simulink model "open_phase_model"  (R2024b)
settings: Solver=ode45  StartTime=0.0  StopTime=0.1  RelTol=1e-3  EnableMultiTasking=on
values from neighbouring files (symbols this model uses):
  load_P = 40e3    (= 40000)    [main.m]
  load_P1 = load_P * 0.3    (= 12000)    [main.m]
  load_P2 = load_P * 0.3    (= 12000)    [main.m]
  load_P3 = load_P * 0.3    (= 12000)    [main.m]
undefined symbols (not defined in the file or in its folder): D1, Delta
libraries: spsFourierLib x6, spsThreePhaseVIMeasurementLib x4, spsRMSLib x4, spsParallelRLCLoadLib x3, spsSequenceAnalyzerLib x2, spsThreePhaseTransformerTwoWindingsLib x2, spsBreakerLib x1, spsThreePhaseSourceLib x1, spsGroundLib x1, spsThreePhasePISectionLineLib x1, spsThreePhaseParallelRLCLoadLib x1, spspowerguiLib x1
settings Model: Creator=jp536285  LastModifiedBy=ahmed
settings SolverCC: AlgebraicLoopSolver=TrustRegion
settings DataIOCC: LimitDataPoints=on  SaveFormat=Array  ReturnWorkspaceOutputs=off
settings OptimizationCC: LifeSpan=inf
settings DebuggingCC: UnderspecifiedInitializationDetection=Classic  MergeDetectMultiDrivingBlocksExec=none  SolverPrmCheckMsg=warning  StateNameClashWarn=warning  SFUnexpectedBacktrackingDiag=warning  SFNoUnconditionalDefaultTransitionDiag=warning  SFExecutionAtInitializationDiag=none  ArithmeticOperatorsInVariantConditions=warning
settings HardwareCC: ProdBitPerPointer=32  ProdBitPerSizeT=32  ProdBitPerPtrDiffT=32  ProdLargestAtomicFloat=None  ProdIntDivRoundTo=Undefined  ProdEndianess=Unspecified  ProdWordSize=32  ProdHWDeviceType=32-bit Generic
settings ModelReferenceCC: PropagateSignalLabelsOutOfModel=off
settings SFSimCC: SimUseLocalCustomCode=off  CustomCodeUndefinedFunction=UseInterfaceOnly
settings RTWCC: RTWUseLocalCustomCode=off  GPUComputeCapability=3.5
settings CodeAppCC: StateflowObjectComments=on
settings GRTTargetCC: TargetLangStandard=C89/C90 (ANSI)
settings ConfigComp: CovMetricSettings=dw  CovSaveCumulativeToWorkspaceVar=on  CovSaveSingleToWorkspaceVar=on  CovExternalEMLEnable=off
settings SimscapeCC: SimscapeNormalizeSystem=off  SimscapeLogOpenViewer=on

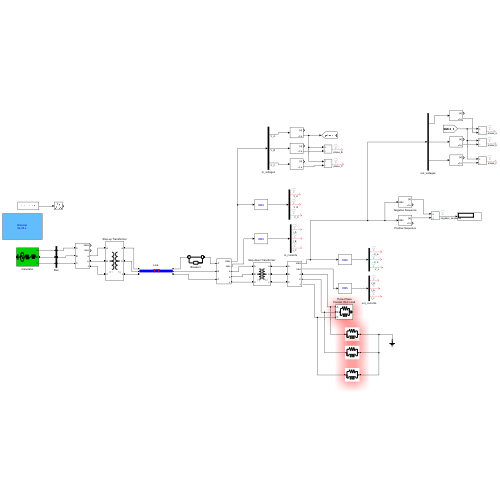
[thumbnail: Simulink's stored preview of the top-level diagram]
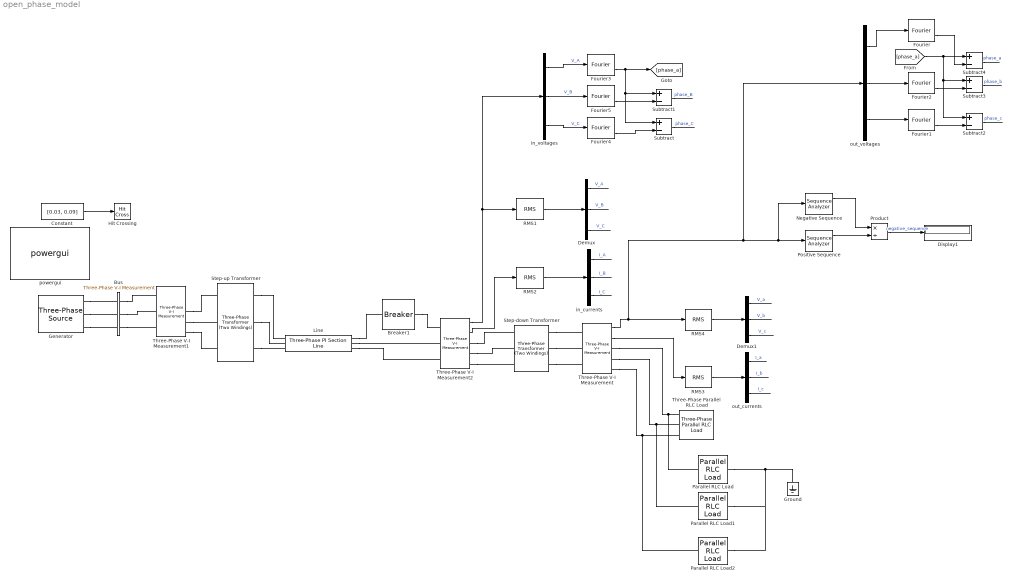
== system open_phase_model ==
  Breaker1 : spsBreakerLib/Breaker  InitialState=1  SwitchingTimes=[3/60]  External=off  BreakerResistance=0.01  SnubberResistance=1e6  SnubberCapacitance=inf  Measurements=None  MoreParameters=on  NoBreakLoop=off
  Bus : spsThreePhaseVIMeasurementLib/Three-Phase V-I Measurement  VoltageMeasurement=phase-to-ground  SetLabelV=on  LabelV=Vabc_3  Vpu=on  VpuLL=off  CurrentMeasurement=yes  SetLabelI=on  LabelI=Iabc_3  Ipu=on  Pbase=100e6  Vbase=13.8e3  OutputType=Complex  PhasorSimulation=off  PSBequivalent=0
  Constant : Constant  Value=[0.03, 0.09]
  Demux : Demux  Outputs=3
  Demux1 : Demux  Outputs=3
  Display1 : Display
  Fourier{,1..5} (6 alike) : spsFourierLib/Fourier  Freq=60  n=1  InInit=[0, 0]  Ts=0
  Generator : spsThreePhaseSourceLib/Three-Phase Source  InternalConnection=Yg  VoltagePhases=off  Voltage=13.8e3  PhaseAngle=0  Voltage_phases=[25e3 25e3 25e3]/sqrt(3)  PhaseAngles_phases=[0 -120 +120]  Frequency=60  NonIdealSource=on  SpecifyImpedance=on  Resistance=0.529  Inductance=0.0140  ShortCircuitLevel=1280e6  BaseVoltage=13.8e3  XRratio=100000  BusType=PV  Pref=85000000  Qref=0  Prefabc=[10e3, 10e3, 10e3]  Qrefabc=[0, 0, 0]  Qmin=-inf  Qmax=inf
  Ground : spsGroundLib/Ground  LConnTagsString=a
  Hit Crossing : HitCross
  Line : spsThreePhasePISectionLineLib/Three-Phase PI Section Line  LConnTagsString=a|b|c  RConnTagsString=A|B|C  Length=10  Frequency=60  Resistances=[ 0.062951 0.15737]  Inductances="[ 1.414e-3  3.53e-3]"  Capacitances=[10.47e-9 6.15e-9]  mask(Three-Phase PI Section Line){}
      mask Display:
      | % This is a new mask on top of the base mask.
      | % Use "View base mask" link below to see the base mask.
      | patch([0.0 0.0 1 1 0.0 0.0 ],[0.4 0.7 0.7 0.4 0.4 0.7],[0 0 1]);
      | patch([0.4 0.4 0.42 0.42],[0.4 0.75 0.75 0.4],[1 0 0]);
      | patch([0.38 0.38 0.57 0.57],[0.7 0.75 0.75 0.7],[1 0 0]);
      | patch([0.53 0.53 0.55 0.55],[0.4 0.75 0.75 0.4],[1 0 0]);
  Negative Sequence : spsSequenceAnalyzerLib/Sequence Analyzer  Freq=60  n=1  seq=Negative  InInit=[1, 0]  Ts=0
      settings: LibrarySourceBlock=sps_lib/Sensors and Measurements/Sequence Analyzer
  Parallel RLC Load : spsParallelRLCLoadLib/Parallel RLC Load  LConnTagsString=a  RConnTagsString=__new0  NominalVoltage=13.8e3/sqrt(3)  NominalFrequency=60  ActivePower=load_P1  InductivePower=load_P1 * 0.75  CapacitivePower=0  Setx0=off  InitialVoltage=0  SetiL0=off  InitialCurrent=0  Measurements=None  LoadType=constant Z
      settings: AttributesFormatString=\n  LibrarySourceBlock=sps_lib/Passives/Parallel RLC Load
  Parallel RLC Load1 : spsParallelRLCLoadLib/Parallel RLC Load  LConnTagsString=a  RConnTagsString=__new0  NominalVoltage=13.8e3/sqrt(3)  NominalFrequency=60  ActivePower=load_P2  InductivePower=load_P2 * 0.75  CapacitivePower=0  Setx0=off  InitialVoltage=0  SetiL0=off  InitialCurrent=0  Measurements=None  LoadType=constant Z
      settings: AttributesFormatString=\n  LibrarySourceBlock=sps_lib/Passives/Parallel RLC Load
  Parallel RLC Load2 : spsParallelRLCLoadLib/Parallel RLC Load  LConnTagsString=a  RConnTagsString=__new0  NominalVoltage=13.8e3/sqrt(3)  NominalFrequency=60  ActivePower=load_P3  InductivePower=load_P3 * 0.75  CapacitivePower=0  Setx0=off  InitialVoltage=0  SetiL0=off  InitialCurrent=0  Measurements=None  LoadType=constant Z
      settings: AttributesFormatString=\n  LibrarySourceBlock=sps_lib/Passives/Parallel RLC Load
  Positive Sequence : spsSequenceAnalyzerLib/Sequence Analyzer  Freq=60  n=1  seq=Positive  InInit=[1, 0]  Ts=0
      settings: LibrarySourceBlock=sps_lib/Sensors and Measurements/Sequence Analyzer
  Product : Product  Inputs=*/
  RMS{1..4} (4 alike) : spsRMSLib/RMS  TrueRMS=on  Freq=60  RMSInit=120  Ts=0
  Step-down Transformer : spsThreePhaseTransformerTwoWindingsLib/Three-Phase Transformer (Two Windings)  Winding1Connection=Yg  Winding2Connection=Delta (D1)  CoreType=Three-limb core (core-type)  SetSaturation=off  Hysteresis=off  DataFile='hysteresis'  SetInitialFlux=off  Measurements=None  UNITS=pu  NominalPower=[ 100e6 , 60 ]  Winding1=[ 230e3 , 1e-6 , 0 ]  Winding2=[ 13.8e3 , 1e-6, 0.0586 ]  Rm=500  Lm=500  L0=0.5  Saturation=[ 0,0 ; 0.0024,1.2 ; 1.0,1.52 ]  InitialFluxes=[ 0.8 , -0.8 , 0.7 ]  BreakLoop=off  DiscreteSolver=Trapezoidal iterative  DataType=off  TransfoNumber=1
  Step-up Transformer : spsThreePhaseTransformerTwoWindingsLib/Three-Phase Transformer (Two Windings)  Winding1Connection=Delta (D1)  Winding2Connection=Yg  CoreType=Three single-phase transformers  SetSaturation=off  Hysteresis=off  DataFile='hysteresis'  SetInitialFlux=off  Measurements=None  UNITS=pu  NominalPower=[ 100e6 , 60 ]  Winding1=[ 13.8e3 , 1e-6 , 0 ]  Winding2=[ 230e3 , 1e-6, 0.0586 ]  Rm=500  Lm=500  L0=0.5  Saturation=[ 0,0 ; 0.0024,1.2 ; 1.0,1.52 ]  InitialFluxes=[ 0.8 , -0.8 , 0.7 ]  BreakLoop=off  DiscreteSolver=Trapezoidal iterative  DataType=off  TransfoNumber=1
  Subtract{,1..4} (5 alike) : Sum  Inputs=+-
  Three-Phase Parallel  RLC Load : spsThreePhaseParallelRLCLoadLib/Three-Phase Parallel RLC Load  LConnTagsString=A|B|C  Configuration=Y (grounded)  NominalVoltage=13800  Vabc=[1e3 1e3 1e3]  Vabcp=[1e3 1e3 1e3]  NominalFrequency=60  UnbalancedPower=off  ActivePower=load_P  InductivePower=load_P * 0.75  CapacitivePower=0  Pabc=[10e3 9e3 11e3]  QLabc=[100 90 110]  QCabc=[100 90 110]  Pabcp=[10e3 9e3 11e3]  QLabcp=[100 90 110]  QCabcp=[100 90 110]  Measurements=None  LoadType=constant PQ
  Three-Phase V-I Measurement : spsThreePhaseVIMeasurementLib/Three-Phase V-I Measurement  VoltageMeasurement=phase-to-ground  SetLabelV=off  LabelV=Vabc  Vpu=off  VpuLL=off  CurrentMeasurement=yes  SetLabelI=off  LabelI=Iabc  Ipu=off  Pbase=100e6  Vbase=500e3  OutputType=Complex  PhasorSimulation=off  PSBequivalent=0
  Three-Phase V-I Measurement1 : spsThreePhaseVIMeasurementLib/Three-Phase V-I Measurement  VoltageMeasurement=phase-to-ground  SetLabelV=off  LabelV=Vabc  Vpu=off  VpuLL=off  CurrentMeasurement=yes  SetLabelI=off  LabelI=Iabc  Ipu=off  Pbase=100e6  Vbase=500e3  OutputType=Complex  PhasorSimulation=off  PSBequivalent=0
  Three-Phase V-I Measurement2 : spsThreePhaseVIMeasurementLib/Three-Phase V-I Measurement  VoltageMeasurement=phase-to-ground  SetLabelV=off  LabelV=Vabc  Vpu=off  VpuLL=off  CurrentMeasurement=yes  SetLabelI=off  LabelI=Iabc  Ipu=off  Pbase=100e6  Vbase=500e3  OutputType=Complex  PhasorSimulation=off  PSBequivalent=0
  in_currents : Demux  Outputs=3
  in_voltages : Demux  Outputs=3
  out_currents : Demux  Outputs=3
  out_voltages : Demux  Outputs=3
  powergui : spspowerguiLib/powergui  Priority=1  SimulationMode=Discrete  SampleTime=50e-6  frequency=60  Iterations=50  frequencyindice=60  Pbase=10e7  ErrMax=1e-05  UnitsV=kV  UnitsW=MW  buscounter=0  FunctionMessages=off  echomessages=off  EnableUseOfTLC=off  CurrentSourceSwitches=on  DisableSnubberDevices=off  DisableRonSwitches=off  DisableVfSwitches=off  DisplayEquations=off  AutomaticDiscreteSolvers=off  SolverType=Tustin  Interpol=off  ExternalGateDelay=off  methode=off  Ts=0  x0status=blocks  SPID=off  SwTol=0  HookPort=off  NonlinearTolerance=1e-4  nMaxIteration=100  ContinueOnMaxIteration=off  RestoreLinks=warning  ResistiveCurrentMeasurement=off  Frange=[0:2:500]  Ylog=off  Xlog=on  ShowGrid=off  save=off  variable=ZData  structure=0  ZoomFFT=off  StartTime=0.0  cycles=1  DisplayStyle=1  fundamental=60  FreqAxis=off  MaxFrequency=1000  frequencyindicesteady=1  RmsSteady=1  display=off
  wires:
  Constant/1 -> Hit Crossing/1
  Fourier/2 -> Subtract4/2
  Three-Phase V-I Measurement/2 -> RMS3/1
  Three-Phase V-I Measurement2/1 -> in_voltages/1, RMS1/1
  Fourier3/2 -> [phase_a], Subtract/1, Subtract1/1
  Three-Phase V-I Measurement2/2 -> RMS2/1
  in_voltages/2 -> Fourier5/1  "V_B"
  out_voltages/1 -> Fourier/1
  out_voltages/2 -> Fourier2/1
  in_voltages/3 -> Fourier4/1  "V_C"
  in_voltages/1 -> Fourier3/1  "V_A"
  Positive Sequence/1 -> Product/2
  RMS2/1 -> in_currents/1
  Fourier5/2 -> Subtract1/2
  Fourier4/2 -> Subtract/2
  Three-Phase V-I Measurement/1 -> Negative Sequence/1, Positive Sequence/1, out_voltages/1, RMS4/1
  Negative Sequence/1 -> Product/1
  out_voltages/3 -> Fourier1/1
  RMS3/1 -> out_currents/1
  Product/1 -> Display1/1  "negative_sequence"
  [phase_a] -> Subtract3/1, Subtract2/1, Subtract4/1
  Fourier2/2 -> Subtract3/2
  Fourier1/2 -> Subtract2/2
  RMS1/1 -> Demux/1
  Demux/1 -> ?  "V_A"
  Demux/2 -> ?  "V_B"
  Demux/3 -> ?  "V_C"
  RMS4/1 -> Demux1/1
  Demux1/1 -> ?  "V_a"
  Demux1/2 -> ?  "V_b"
  Demux1/3 -> ?  "V_c"
  out_currents/1 -> ?  "I_a"
  out_currents/2 -> ?  "I_b"
  out_currents/3 -> ?  "I_c"
  in_currents/1 -> ?  "I_A"
  in_currents/2 -> ?  "I_B"
  in_currents/3 -> ?  "I_C"
  Subtract4/1 -> ?  "phase_a"
  Subtract3/1 -> ?  "phase_b"
  Subtract2/1 -> ?  "phase_c"
  Subtract1/1 -> ?  "phase_B"
  Subtract/1 -> ?  "phase_C"
  connections:
  Generator/RConn2 -- Bus/RConn2
  Step-up Transformer/RConn1 -- Line/RConn1
  Generator/RConn1 -- Bus/RConn1
  Three-Phase V-I Measurement/RConn1 -- Parallel RLC Load/LConn1 -- Three-Phase Parallel  RLC Load/LConn1
  Bus/LConn1 -- Three-Phase V-I Measurement1/LConn1
  Line/LConn2 -- Three-Phase V-I Measurement2/LConn2
  Generator/RConn3 -- Bus/RConn3
  Three-Phase V-I Measurement1/RConn1 -- Step-up Transformer/LConn1
  Three-Phase V-I Measurement2/RConn2 -- Step-down Transformer/LConn2
  Three-Phase V-I Measurement1/RConn3 -- Step-up Transformer/LConn3
  Bus/LConn2 -- Three-Phase V-I Measurement1/LConn2
  Bus/LConn3 -- Three-Phase V-I Measurement1/LConn3
  Three-Phase V-I Measurement2/RConn1 -- Step-down Transformer/LConn1
  Three-Phase V-I Measurement1/RConn2 -- Step-up Transformer/LConn2
  Step-up Transformer/RConn2 -- Line/RConn2
  Step-up Transformer/RConn3 -- Line/RConn3
  Line/LConn1 -- Breaker1/LConn1
  Line/LConn3 -- Three-Phase V-I Measurement2/LConn3
  Breaker1/RConn1 -- Three-Phase V-I Measurement2/LConn1
  Three-Phase V-I Measurement/RConn2 -- Parallel RLC Load1/LConn1 -- Three-Phase Parallel  RLC Load/LConn2
  Three-Phase V-I Measurement2/RConn3 -- Step-down Transformer/LConn3
  Step-down Transformer/RConn1 -- Three-Phase V-I Measurement/LConn1
  Step-down Transformer/RConn2 -- Three-Phase V-I Measurement/LConn2
  Step-down Transformer/RConn3 -- Three-Phase V-I Measurement/LConn3
  Three-Phase V-I Measurement/RConn3 -- Parallel RLC Load2/LConn1 -- Three-Phase Parallel  RLC Load/LConn3
  Parallel RLC Load/RConn1 -- Parallel RLC Load2/RConn1 -- Parallel RLC Load1/RConn1 -- Ground/LConn1
